simulink model "feedback"  (R2017b)
settings: Solver=ode3  StartTime=0.0  StopTime=1  RelTol=1e-3
libraries: powerlib x30, powerlib_meascontrol x2, simulink x1
settings Model: Creator=user  LastModifiedBy=HP
settings DataIOCC: ReturnWorkspaceOutputs=on
settings SFSimCC: SimUseLocalCustomCode=on
settings RTWCC: RTWUseLocalCustomCode=on

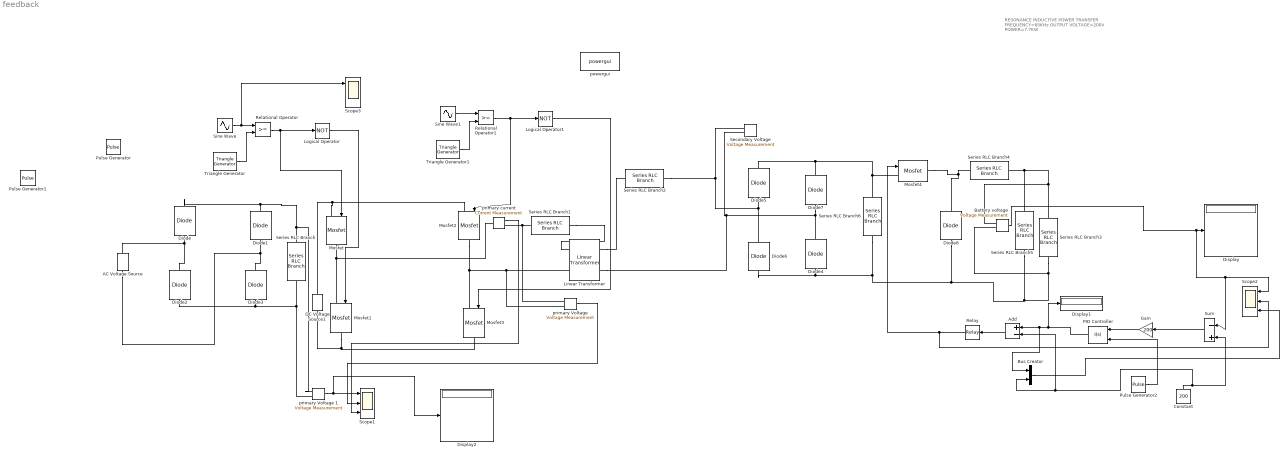
== system feedback ==
  note: RESONANCE INDUCTIVE POWER TRANSFER
      |
      | FREQUENCY=85KHz
      | OUTPUT VOLTAGE=200V
      | POWER=7.7KW
  " Battery voltage " : powerlib/Measurements/Voltage Measurement  PhasorSimulation=off  OutputType=Complex  PSBequivalent=0
  AC Voltage Source : powerlib/Electrical Sources/AC Voltage Source  Amplitude=16.97056275  Phase=0  Frequency=50  SampleTime=0  Measurements=Voltage  BusType=swing  Pref=10e3  Qref=0  Qmin=-inf  Qmax=+inf
  Add : Sum  Inputs=+-
  Bus Creator : BusCreator  Inputs=2
  Constant : Constant  Value=200
  DC Voltage Source1 : powerlib/Electrical Sources/DC Voltage Source  Amplitude=15  Measurements=Voltage
  Diode{,1..8} (9 alike) : powerlib/Power Electronics/Diode  Ron=0.001  Lon=0  Vf=0.8  IC=0  UseSnubber=0  Rs=500  Cs=250e-9  Measurements=off
  Display : Display
  Display1 : Display
  Display2 : Display
      settings: Decimation=3
  Gain : Gain  Gain=200
  Linear Transformer : powerlib/Elements/Linear Transformer  UNITS=SI  NominalPower=[ 7700 85000 ]  winding1=[500 0.068 0.0001608]  winding2=[500 0.063 0.00014006]  ThreeWindings=off  winding3=[3.15e+05 0.7938 0.084222]  RmLm=[1.0805e+06 2866]  Measurements=All voltages and currents  DataType=on
  Logical Operator : Logic  Operator=NOT  AllPortsSameDT=off  OutDataTypeStr=boolean
  Logical Operator1 : Logic  Operator=NOT  AllPortsSameDT=off  OutDataTypeStr=boolean
  Mosfet{,1..4} (5 alike) : powerlib/Power Electronics/Mosfet  Ron=0.1  Lon=0  Rd=0.01  Vfd=0  IC=0  Rs=1e5  Cs=inf  Measurements=off
  PID Controller : simulink/Continuous/PID Controller  Controller=I  Form=Parallel  TimeDomain=Continuous-time  SampleTime=-1  IntegratorMethod=Forward Euler  FilterMethod=Forward Euler  ControllerParametersSource=internal  P=-1.5  I=340000  D=0  UseFilter=on  N=100  TunerSelectOption=Transfer Function Based (PID Tuner App)  InitialConditionSource=internal  InitialConditionForIntegrator=0  InitialConditionForFilter=0  DifferentiatorICPrevScaledInput=0  ExternalReset=falling  TrackingMode=off  Kt=1  LimitOutput=off  UpperSaturationLimit=1  LowerSaturationLimit=0  LinearizeAsGain=on  AntiWindupMode=none  Kb=1  POutMin=[]  POutMax=[]  IOutMin=[]  IOutMax=[]  DOutMin=[]  DOutMax=[]  NOutMin=[]  NOutMax=[]  SumOutMin=[]  SumOutMax=[]  SaturationOutMin=[]  SaturationOutMax=[]  PParamMin=[]  PParamMax=[]  IParamMin=[]  IParamMax=[]  DParamMin=[]  DParamMax=[]  NParamMin=[]  NParamMax=[]  KbParamMin=[]  KbParamMax=[]  KtParamMin=[]  KtParamMax=[]  KbOutMin=[]  KbOutMax=[]  KtOutMin=[]  KtOutMax=[]  IntegratorOutMin=[]  IntegratorOutMax=[]  FilterOutMin=[]  FilterOutMax=[]  SumI1OutMin=[]  SumI1OutMax=[]  SumI2OutMin=[]  SumI2OutMax=[]  SumI3OutMin=[]  SumI3OutMax=[]  SumDOutMin=[]  SumDOutMax=[]  DifferentiatorOutMin=[]  DifferentiatorOutMax=[]  FilterDiffOutCoefMin=[]  FilterDiffOutCoefMax=[]  ReciprocalOutMin=[]  ReciprocalOutMax=[]  SumDenOutMin=[]  SumDenOutMax=[]  SumNumOutMin=[]  SumNumOutMax=[]  DivideOutMin=[]  DivideOutMax=[]  IntegratorContinuousStateAttributes=''  IntegratorStateMustResolveToSignalObject=off  IntegratorRTWStateStorageClass=Auto  FilterContinuousStateAttributes=''  FilterStateMustResolveToSignalObject=off  FilterRTWStateStorageClass=Auto  InitialConditionSetting=State (most efficient)
  Pulse Generator : DiscretePulseGenerator  PulseType=Time based  Period=1/85000  PulseWidth=50  PhaseDelay=5.88235294e-6
  Pulse Generator1 : DiscretePulseGenerator  PulseType=Time based  Period=1/85000  PulseWidth=50
  Pulse Generator2 : DiscretePulseGenerator  PulseType=Time based  Period=1/85000  PulseWidth=50
  Relational Operator : RelationalOperator  OutDataTypeStr=boolean  RndMeth=Simplest
  Relational Operator1 : RelationalOperator  OutDataTypeStr=boolean  RndMeth=Simplest
  Relay : Relay
  Scope1 : Scope  NumInputPorts=3
  Scope2 : Scope  NumInputPorts=3
  Scope3 : Scope  NumInputPorts=3
  "Secondary Voltage " : powerlib/Measurements/Voltage Measurement  PhasorSimulation=off  OutputType=Complex  PSBequivalent=0
  Series RLC Branch : powerlib/Elements/Series RLC Branch  LConnTagsString=__new0  RConnTagsString=__new0  BranchType=C  Resistance=1  Inductance=1e-3  SetiL0=off  InitialCurrent=0  Capacitance=10e-6  Setx0=off  InitialVoltage=0  Measurements=None
  Series RLC Branch1 : powerlib/Elements/Series RLC Branch  LConnTagsString=__new0  RConnTagsString=__new0  BranchType=C  Resistance=1  Inductance=1e-3  SetiL0=off  InitialCurrent=0  Capacitance=2.217e-8  Setx0=off  InitialVoltage=0  Measurements=None
  Series RLC Branch2 : powerlib/Elements/Series RLC Branch  LConnTagsString=__new0  RConnTagsString=__new0  BranchType=C  Resistance=1  Inductance=1e-3  SetiL0=off  InitialCurrent=0  Capacitance=2.545e-8  Setx0=off  InitialVoltage=0  Measurements=None
  Series RLC Branch3 : powerlib/Elements/Series RLC Branch  LConnTagsString=__new0  RConnTagsString=__new0  BranchType=R  Resistance=4.210750489  Inductance=.0021  SetiL0=off  InitialCurrent=0  Capacitance=1e-6  Setx0=off  InitialVoltage=0  Measurements=Branch voltage
  Series RLC Branch4 : powerlib/Elements/Series RLC Branch  LConnTagsString=__new0  RConnTagsString=__new0  BranchType=L  Resistance=1  Inductance=.0021  SetiL0=off  InitialCurrent=0  Capacitance=1e-6  Setx0=off  InitialVoltage=0  Measurements=None
  Series RLC Branch5 : powerlib/Elements/Series RLC Branch  LConnTagsString=__new0  RConnTagsString=__new0  BranchType=C  Resistance=1  Inductance=1e-3  SetiL0=off  InitialCurrent=0  Capacitance=5.882e-6  Setx0=off  InitialVoltage=0  Measurements=None
  Series RLC Branch6 : powerlib/Elements/Series RLC Branch  LConnTagsString=__new0  RConnTagsString=__new0  BranchType=C  Resistance=1  Inductance=1e-3  SetiL0=off  InitialCurrent=0  Capacitance=49.19e-6  Setx0=off  InitialVoltage=0  Measurements=None
  Sine Wave : Sin  Frequency=534070  SampleTime=0
  Sine Wave1 : Sin  Frequency=534070  Phase=180  SampleTime=0
  Sum : Sum  Inputs=|-+
  Triangle Generator : powerlib_meascontrol/Pulse & Signal Generators/Triangle Generator  Freq=1700e3  Phase=0  Ts=0
  Triangle Generator1 : powerlib_meascontrol/Pulse & Signal Generators/Triangle Generator  Freq=1700e3  Phase=0  Ts=0
  powergui : powerlib/powergui  Priority=1  SimulationMode=Discrete  SampleTime=1e-7  frequency=60  Iterations=50  frequencyindice=0  Pbase=100e6  ErrMax=1e-4  UnitsV=kV  UnitsW=MW  buscounter=0  FunctionMessages=off  echomessages=off  EnableUseOfTLC=off  CurrentSourceSwitches=off  DisableSnubberDevices=off  DisableRonSwitches=off  DisableVfSwitches=off  DisplayEquations=off  AutomaticDiscreteSolvers=off  SolverType=Tustin/Backward Euler (TBE)  Interpol=off  ExternalGateDelay=off  methode=off  Ts=100  x0status=blocks  SPID=on  SwTol=0  HookPort=off  NonlinearTolerance=1e-4  nMaxIteration=100  ContinueOnMaxIteration=off  RestoreLinks=warning  ResistiveCurrentMeasurement=off  Frange=[0:2:500]  Ylog=off  Xlog=on  ShowGrid=off  save=off  variable=ZData  structure=0  ZoomFFT=off  StartTime=0.0  cycles=1  DisplayStyle=1  fundamental=60  FreqAxis=off  MaxFrequency=1000  frequencyindicesteady=1  RmsSteady=1  display=off
  "primary Voltage " : powerlib/Measurements/Voltage Measurement  PhasorSimulation=off  OutputType=Complex  PSBequivalent=0
  primary Voltage 1 : powerlib/Measurements/Voltage Measurement  PhasorSimulation=off  OutputType=Complex  PSBequivalent=0
  primary current : powerlib/Measurements/Current Measurement  PhasorSimulation=off  OutputType=Complex  PSBequivalent=0
  wires:
  Constant/1 -> Add/2, Bus Creator/2, Sum/2
  Pulse Generator2/1 -> PID Controller/2
  Add/1 -> Relay/1
  Gain/1 -> PID Controller/1
  " Battery voltage "/1 -> Scope2/1, Sum/1, Display/1
  PID Controller/1 -> Display1/1, Add/1, Bus Creator/1
  Relay/1 -> Scope2/2, Mosfet4/1
  Bus Creator/1 -> Scope2/3
  Sum/1 -> Gain/1
  primary Voltage 1/1 -> Display2/1, Scope1/1
  Sine Wave/1 -> Scope3/1, Relational Operator/1
  Triangle Generator/1 -> Relational Operator/2
  Relational Operator/1 -> Mosfet/1, Logical Operator/1
  Logical Operator/1 -> Mosfet1/1
  Sine Wave1/1 -> Relational Operator1/1
  Triangle Generator1/1 -> Relational Operator1/2
  Relational Operator1/1 -> Mosfet2/1, Logical Operator1/1
  Logical Operator1/1 -> Mosfet3/1
  "primary Voltage "/1 -> Scope1/2
  primary current/1 -> Scope1/3
  connections:
  Diode2/RConn1 -- AC Voltage Source/RConn1 -- Diode/LConn1
  Diode3/RConn1 -- AC Voltage Source/LConn1 -- Diode1/LConn1
  Mosfet1/LConn1 -- primary current/LConn1 -- Mosfet/RConn1
  Mosfet2/RConn1 -- "primary Voltage "/LConn2 -- Linear Transformer/LConn2 -- Mosfet3/LConn1
  Series RLC Branch1/LConn1 -- Linear Transformer/LConn1
  Linear Transformer/RConn1 -- Series RLC Branch2/LConn1
  Diode6/RConn1 -- "Secondary Voltage "/LConn1 -- Series RLC Branch2/RConn1 -- Diode5/LConn1
  Linear Transformer/RConn2 -- Diode4/RConn1 -- Diode7/LConn1 -- "Secondary Voltage "/LConn2
  Diode7/RConn1 -- Series RLC Branch6/LConn1 -- Mosfet4/LConn1 -- Diode5/RConn1
  Diode6/LConn1 -- Series RLC Branch6/RConn1 -- " Battery voltage "/LConn2 -- Series RLC Branch3/RConn1 -- Series RLC Branch5/RConn1 -- Diode8/LConn1 -- Diode4/LConn1
  Mosfet4/RConn1 -- Diode8/RConn1 -- Series RLC Branch4/LConn1
  Series RLC Branch5/LConn1 -- " Battery voltage "/LConn1 -- Series RLC Branch3/LConn1 -- Series RLC Branch4/RConn1
  Series RLC Branch1/RConn1 -- primary current/RConn1 -- "primary Voltage "/LConn1
  Diode/RConn1 -- primary Voltage 1/LConn1 -- Series RLC Branch/LConn1 -- Diode1/RConn1
  Diode2/LConn1 -- primary Voltage 1/LConn2 -- Series RLC Branch/RConn1 -- Diode3/LConn1
  Mosfet/LConn1 -- Mosfet2/LConn1 -- DC Voltage Source1/RConn1
  Mosfet1/RConn1 -- DC Voltage Source1/LConn1 -- Mosfet3/RConn1
